simulink model "MATE_SimpleRLC"  (R2024b)
settings: Solver=FixedStepDiscrete  StartTime=0.0  StopTime=0.03  FixedStep=Ts  RelTol=1e-3  AbsTol=1e-2
PostLoadFcn:
  | Ts = 30e-6;
InitFcn:
  | Ts = 30e-6;
StartFcn:
  | Ts=100e-6;
undefined symbols (not defined in the file): MATE, MATE1ph, MATERT, simetran
libraries: fl_lib x17, nesl_utility x9, ee_lib x4, simetranss x2
settings Model: ARTEMISmethode_block_infos=$$__separator__$$  ModifiedByFormat=Kyle  Creator=Kyle Diller  LastModifiedBy=Kyle
settings SolverCC: AutoScaleAbsTol=off  AlgebraicLoopSolver=TrustRegion
settings DataIOCC: SaveFormat=Array  SignalLoggingSaveFormat=ModelDataLogs  ReturnWorkspaceOutputs=off  TimeSaveName=t  OutputSaveName=y  SignalLoggingName=sigsOut
settings OptimizationCC: BlockReduction=off  BooleanDataType=off  ExpressionDepthLimit=2147483647  InitFltsAndDblsToZero=on  LifeSpan=inf
settings DebuggingCC: AlgebraicLoopMsg=none  SaveWithParameterizedLinksMsg=none  UnderspecifiedInitializationDetection=Classic  MergeDetectMultiDrivingBlocksExec=none  SignalResolutionControl=TryResolveAllWithWarning  MultiTaskDSMMsg=warning  MultiTaskCondExecSysMsg=none  FcnCallInpInsideContextMsg=warning  UnconnectedInputMsg=warning  UnconnectedOutputMsg=warning  UnconnectedLineMsg=warning  AllowSymbolicDim=off  StateNameClashWarn=warning  SFUnexpectedBacktrackingDiag=warning  SFNoUnconditionalDefaultTransitionDiag=warning  SFExecutionAtInitializationDiag=none  ArithmeticOperatorsInVariantConditions=warning
settings HardwareCC: ProdBitPerPointer=32  ProdBitPerSizeT=32  ProdBitPerPtrDiffT=32  ProdLargestAtomicFloat=None  ProdIntDivRoundTo=Undefined  ProdEndianess=Unspecified  ProdWordSize=32  ProdHWDeviceType=32-bit Generic  TargetUnknown=on
settings ModelReferenceCC: EnableRefExpFcnMdlSchedulingChecks=on  PropagateSignalLabelsOutOfModel=off
settings SFSimCC: SimUseLocalCustomCode=off  CustomCodeUndefinedFunction=UseInterfaceOnly
settings RTWCC: TemplateMakefile=grt_unix.tmf  RTWUseLocalCustomCode=off  GPUComputeCapability=3.5
settings CodeAppCC: StateflowObjectComments=on
settings GRTTargetCC: TargetFcnLib=ansi_tfl_tmw.mat  TargetLangStandard=C89/C90 (ANSI)  CombineOutputUpdateFcns=off  GRTInterface=on
settings ConfigComp: CovMetricSettings=dw  CovSaveCumulativeToWorkspaceVar=on  CovSaveSingleToWorkspaceVar=on  CovExternalEMLEnable=off
settings SimscapeCC: SimscapeNormalizeSystem=off

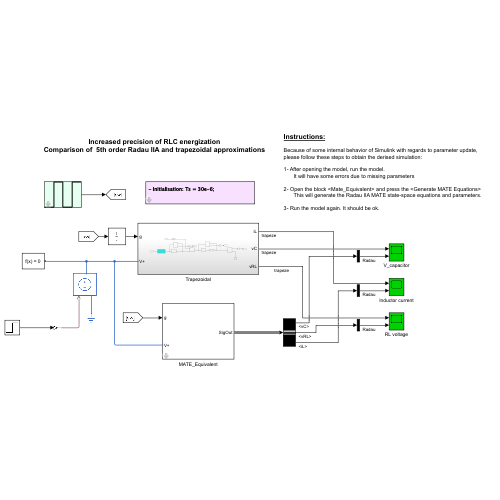
[thumbnail: Simulink's stored preview of the top-level diagram]
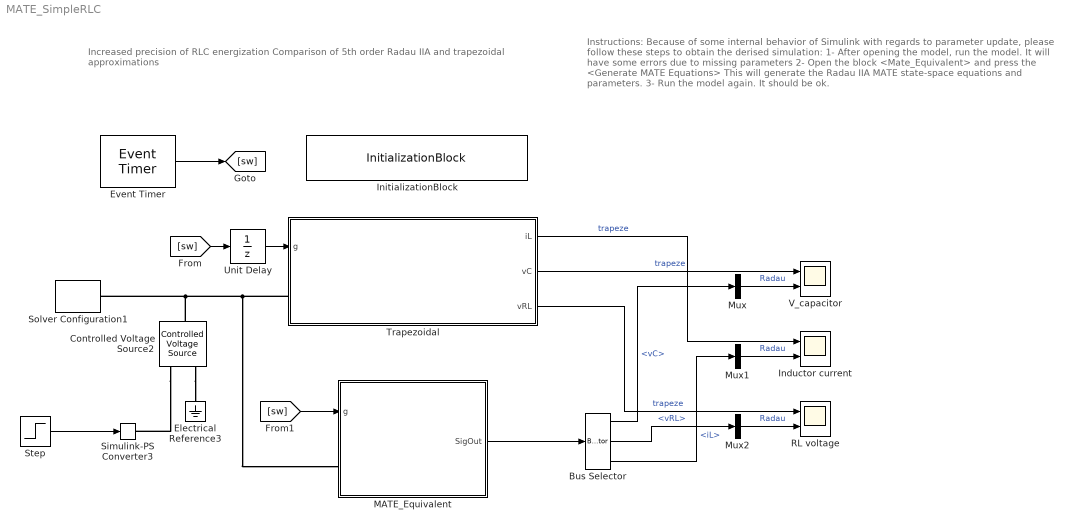
== system MATE_SimpleRLC ==
  note: Instructions:
      |
      | Because of some internal behavior of Simulink with regards to parameter update,
      | please follow these steps to obtain the derised simulation:
      |
      | 1- After opening the model, run the model.
      | It will have some errors due to missing parameters
      |
      | 2- Open the block <Mate_Equivalent> and press the <Generate MATE Equations>
      | This will generate the Radau IIA MATE state-space equations and parameters.
      |
      | 3- Run the model again. It should be ok.
  note: Increased precision of RLC energization
      | Comparison of  5th order Radau IIA and trapezoidal approximations
  Bus Selector : BusSelector  OutputSignals=vC,vRL,iL
  Controlled Voltage Source2 : fl_lib/Electrical/Electrical Sources/Controlled Voltage Source
  Electrical Reference3 : fl_lib/Electrical/Electrical Elements/Electrical Reference
  Event Timer : simetranss/Usefulls/Event Timer  Tag=RTEcontrol_s38shd7k88  is=0 (off)  t=[0.01 0.02 0.03 0.04 ]  Tmax=0.07  Ts=Ts
  Inductor current : Scope  NumInputPorts=2
  InitializationBlock : simetranss/Usefulls/InitializationBlock  InitVar=Ts = 30e-6;  prel=off  posl=on  inif=on
  MATE_Equivalent : Subsystem  mask(MATE object){MATE=MATE, MATERT=MATERT, subsys='MATE_SimpleRLC/Trapezoidal', discmeth=5th order accurate fully-implicit three-stage Runge-Kutta formula (Radau IIA), Tsx=Ts}
      mask prompts: MATE "General MATE data structure name"; MATERT "MATE S-function parameter"; subsys "Reference subsystem for MATE"; discmeth "Discretization"; Tsx "Sample time (s)"
      mask help: The MATE Object contains the MATE solver for mixed nodal and state-space equation of the MATE solution. This is a beta block.
      mask TypeOptions discmeth: Backward Euler | Trapezoidal |  5th order accurate fully-implicit three-stage Runge-Kutta formula (Radau IIA)
      mask DialogControl Control2 Prompt: Generate MATE equations
      mask DialogControl Control2 Callback:
      | block=gcb;
      | maskObj = Simulink.Mask.get(block); % get mask handle
      | Ts = get_param(block, 'value@Tsx'); % retrieve value for Vrated
      | sub = get_param(block, 'value@subsys'); % retrieve value for Vmin_p
      | dd = get_param(block, 'value@discmeth'); % retrieve value for Vmin_p
      | if dd==3
      |     dd=5;
      | end
      | %Tss=get_param(block,'Ts')
      | [MATE, MATERT]= MakeMate2(sub , dd, Ts);
      | assignin("base","MATE",MATE);
      | assignin("base","MATERT",MATERT);
  Mux : Mux  Inputs=1
  Mux1 : Mux  Inputs=1
  Mux2 : Mux  Inputs=1
  RL voltage : Scope  NumInputPorts=2
  Simulink-PS Converter3 : nesl_utility/Simulink-PS Converter  PhysicalDomain=network_engine_domain  SubClassName=ps_input  LeftPortType=input  RightPortType=output  PseudoPeriodic=off  Frequencies=[]  NoiseDistribution=none  NoiseParameters=[]  Unit=1  AffineConversion=off  FilteringAndDerivatives=provide  SimscapeFilterOrder=1  InputFilterTimeConstant=0.001  UdotUserProvided=0
  Solver Configuration1 : nesl_utility/Solver Configuration  PhysicalDomain=network_engine_domain  SubClassName=solver  LeftPortType=input  RightPortType=generic  Tones=[]  Harmonics=[]  SimulateNoise=off  Profile=off  UseLocalSampling=off  EnableSwitchedLinearOptims=on  FrequencyDomain=off  UseCCode=off  RelTol=0.001  AbsTol=1e-06  MinStep=1e-09  ToWorkspace=off  RevertToSquareIcSolve=off  NumHomotopyIterations=100  PhasorMode=off  PhasorModeNumHarmonics=1  ConsistencySolver=NEWTON_FTOL  IndexReductionMethod=DerivativeReplacement  DoDC=off  ResidualTolerance=1e-09  ConsistencyTolSource=GLOBAL  ConsistencyAbsTol=0.001  ConsistencyRelTol=0.001  ConsistencyTolFactor=0.001  UseLocalSolver=on  LocalSolverChoice=NE_TRAPEZOIDAL_ADVANCER  ResolveIndetEquations=on  FunctionEvalNumThread=1  LocalSolverSampleTime=Ts  DoFixedCost=on  MaxNonlinIter=1  MaxModeIter=2  ComputeImpulses=on  ImpulseIterations=2  LinearAlgebra=auto  LinearAlgebraNumThread=0  EquationFormulation=NE_TIME_EF  DelaysMemoryBudget=1024  AutomaticFiltering=on  FilteringTimeConstant=0.001  PartitionStorageMethod=AS_NEEDED  PartitionMemoryBudget=1024  PartitionMethod=ROBUST  MultibodyUseLocalSolver=off  MultibodyLocalSolverChoice=ODE1  MultibodyLocalSolverSampleTime=0.001
  Step : Step  Time=1e-3  SampleTime=0
  Trapezoidal : Subsystem
  Unit Delay : UnitDelay  SampleTime=Ts  HasFrameUpgradeWarning=on
  V_capacitor : Scope  NumInputPorts=2
  wires:
  MATE_Equivalent/1(SigOut) -> Bus Selector/1
  [sw] -> Unit Delay/1
  [sw] -> MATE_Equivalent/1(g)
  Event Timer/1 -> [sw]
  Trapezoidal/3(vRL) -> RL voltage/1  "trapeze"
  Trapezoidal/1(iL) -> Inductor current/1  "trapeze"
  Bus Selector/3 -> Mux1/1  "<iL>"
  Trapezoidal/2(vC) -> V_capacitor/1  "trapeze"
  Bus Selector/1 -> Mux/1  "<vC>"
  Bus Selector/2 -> Mux2/1  "<vRL>"
  Step/1 -> Simulink-PS Converter3/1
  Unit Delay/1 -> Trapezoidal/1(g)
  Mux/1 -> V_capacitor/2  "Radau"
  Mux1/1 -> Inductor current/2  "Radau"
  Mux2/1 -> RL voltage/2  "Radau"
  connections:
  Solver Configuration1/RConn1 -- Trapezoidal/LConn1 -- MATE_Equivalent/LConn1 -- Controlled Voltage Source2/LConn1
  Controlled Voltage Source2/RConn2 -- Electrical Reference3/LConn1
  Controlled Voltage Source2/RConn1 -- Simulink-PS Converter3/RConn1

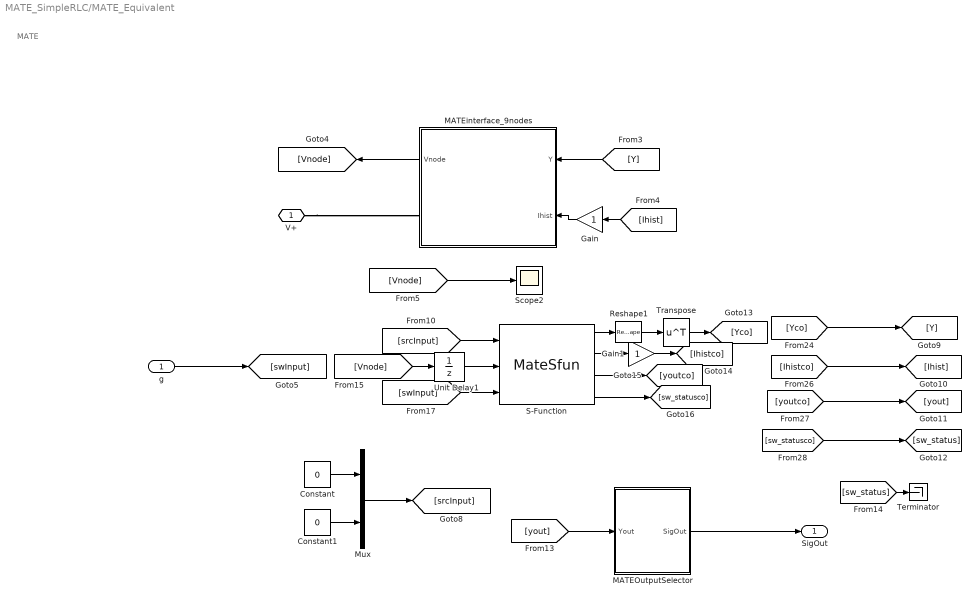
== system MATE_SimpleRLC/MATE_Equivalent ==
  note: MATE
  g : Inport
  Constant : Constant  Value=0
  Constant1 : Constant  Value=0
  Gain : Gain
  Gain1 : Gain
  MATEOutputSelector : Subsystem
  MATEinterface_9nodes : Subsystem
  Mux : Mux  Inputs=2
  Reshape1 : Reshape  OutputDimensionality=Customize  OutputDimensions=[MATE.NumberOfNodes,MATE.NumberOfNodes]
  S-Function : S-Function  FunctionName=MateSfun  Parameters="MATERT.sizes,MATERT.As  ,MATERT.Bs,MATERT.Cs,MATERT.Ds,MATERT.Rsw,MATERT.SwType,MATERT.DISC,MATERT.h,MATERT.U0,MATERT.X0,MATERT.SwitchVf"  SFunctionDeploymentMode=off  EnableBusSupport=off
  Scope2 : Scope
  Terminator : Terminator
  Transpose : Math  Operator=transpose
  Unit Delay1 : UnitDelay  SampleTime=Ts  HasFrameUpgradeWarning=on
  V+ : PMIOPort  Side=Left
  SigOut : Outport
  wires:
  MATEOutputSelector/1(SigOut) -> SigOut/1
  [Vnode] -> Scope2/1
  Mux/1 -> [srcInput]
  g/1 -> [swInput]
  [Yco] -> [Y]
  S-Function/4 -> [sw_statusco]
  [Ihist] -> Gain/1
  [srcInput] -> S-Function/1
  [Ihistco] -> [Ihist]
  Unit Delay1/1 -> S-Function/2
  [swInput] -> S-Function/3
  Reshape1/1 -> Transpose/1
  [Y] -> MATEinterface_9nodes/1(Y)
  [sw_status] -> Terminator/1
  Transpose/1 -> [Yco]
  [yout] -> MATEOutputSelector/1(Yout)
  S-Function/3 -> [youtco]
  [Vnode] -> Unit Delay1/1
  [youtco] -> [yout]
  S-Function/2 -> Gain1/1
  MATEinterface_9nodes/1(Vnode) -> [Vnode]
  S-Function/1 -> Reshape1/1
  [sw_statusco] -> [sw_status]
  Gain/1 -> MATEinterface_9nodes/2(Ihist)
  Gain1/1 -> [Ihistco]
  Constant/1 -> Mux/1
  Constant1/1 -> Mux/2
  connections:
  V+/RConn1 -- MATEinterface_9nodes/RConn1

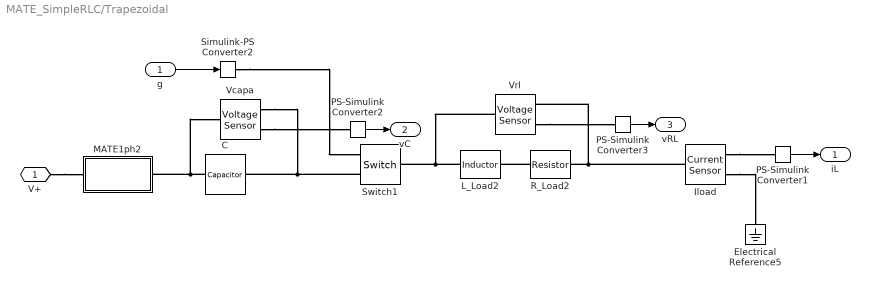
== system MATE_SimpleRLC/Trapezoidal ==
  g : Inport
  C : fl_lib/Electrical/Electrical Elements/Capacitor  c=1e-6 F  r=0 Ohm  g=0 1/Ohm  i_specify=off  i_priority=None  i=0 A  i_nominal_specify=off  i_nominal_value=1  i_nominal_unit=A  v_specify=on  v_priority=None  v=0 V  v_nominal_specify=off  v_nominal_value=1  v_nominal_unit=V  vc_specify=off  vc_priority=High  vc=0 V  vc_nominal_specify=off  vc_nominal_value=1  vc_nominal_unit=V
      settings: AttributesFormatString=%<c> %<c_unit>
  Electrical Reference5 : fl_lib/Electrical/Electrical Elements/Electrical Reference
  Iload : fl_lib/Electrical/Electrical Sensors/Current Sensor
  L_Load2 : fl_lib/Electrical/Electrical Elements/Inductor  l=3e-3 H  r=0 Ohm  g=0 1/Ohm  i_specify=on  i_priority=None  i=0 A  i_nominal_specify=off  i_nominal_value=1  i_nominal_unit=A  v_specify=off  v_priority=None  v=0 V  v_nominal_specify=off  v_nominal_value=1  v_nominal_unit=V  i_L_specify=off  i_L_priority=High  i_L=0 A  i_L_nominal_specify=off  i_L_nominal_value=1  i_L_nominal_unit=A
      settings: AttributesFormatString=%<l> %<l_unit>
  MATE1ph2 : Subsystem  AncestorBlock=simetran/MATE1ph  mask(MATE Node (1ph)){bn=1, conty=Single-Phase, it=auto, Rse=1e-4, Rsh=1e9}
      mask prompts: bn "MATE node number"; conty "Connection"; it "Interface type"; Rse "Series resistance (Ohms)"; Rsh "Shunt resistance (Ohms)"
      mask help:
      | MATE interface for single phase SimScape model.
      |
      | This block is used to interface a MATE reduced set of block to a main circuit.
      | 'MATE' port must be connected toward the MATE reduced network.
      | 'Main' port must be connected toward the main (unreduced) network)
      settings: AttributesFormatString=# %<bn>
      mask TypeOptions conty: Single-Phase | 3-phase SLD | 3-phase expended
      mask TypeOptions it: auto | Thevenin | Norton
  PS-Simulink Converter1 : nesl_utility/PS-Simulink Converter  PhysicalDomain=network_engine_domain  SubClassName=ps_output  LeftPortType=input  RightPortType=output  PseudoPeriodic=off  Frequencies=[]  VectorFormat=inherit  Unit=inherit  AffineConversion=off
  PS-Simulink Converter2 : nesl_utility/PS-Simulink Converter  PhysicalDomain=network_engine_domain  SubClassName=ps_output  LeftPortType=input  RightPortType=output  PseudoPeriodic=off  Frequencies=[]  VectorFormat=inherit  Unit=inherit  AffineConversion=off
  PS-Simulink Converter3 : nesl_utility/PS-Simulink Converter  PhysicalDomain=network_engine_domain  SubClassName=ps_output  LeftPortType=input  RightPortType=output  PseudoPeriodic=off  Frequencies=[]  VectorFormat=inherit  Unit=inherit  AffineConversion=off
  R_Load2 : fl_lib/Electrical/Electrical Elements/Resistor  R=2 Ohm  i_specify=off  i_priority=None  i=0 A  i_nominal_specify=off  i_nominal_value=1  i_nominal_unit=A  v_specify=off  v_priority=None  v=0 V  v_nominal_specify=off  v_nominal_value=1  v_nominal_unit=V
      settings: AttributesFormatString=%<R> %<R_unit>
  Simulink-PS Converter2 : nesl_utility/Simulink-PS Converter  PhysicalDomain=network_engine_domain  SubClassName=ps_input  LeftPortType=input  RightPortType=output  PseudoPeriodic=off  Frequencies=[]  NoiseDistribution=none  NoiseParameters=[]  Unit=1  AffineConversion=off  FilteringAndDerivatives=provide  SimscapeFilterOrder=1  InputFilterTimeConstant=0.001  UdotUserProvided=0
  Switch1 : fl_lib/Electrical/Electrical Elements/Switch  R_closed=0.01 Ohm  G_open=1e-8 1/Ohm  Threshold=0.5  i_specify=off  i_priority=None  i=0 A  i_nominal_specify=off  i_nominal_value=1  i_nominal_unit=A  v_specify=off  v_priority=None  v=0 V  v_nominal_specify=off  v_nominal_value=1  v_nominal_unit=V
  Vcapa : fl_lib/Electrical/Electrical Sensors/Voltage Sensor
  Vrl : fl_lib/Electrical/Electrical Sensors/Voltage Sensor
  V+ : PMIOPort  Side=Left
  iL : Outport
  vC : Outport  Port=2
  vRL : Outport  Port=3
  wires:
  PS-Simulink Converter2/1 -> vC/1
  PS-Simulink Converter1/1 -> iL/1
  g/1 -> Simulink-PS Converter2/1
  PS-Simulink Converter3/1 -> vRL/1
  connections:
  C/RConn1 -- Vcapa/LConn1 -- MATE1ph2/RConn1
  Vcapa/RConn2 -- Switch1/RConn2 -- C/LConn1
  Iload/RConn1 -- PS-Simulink Converter1/LConn1
  Vcapa/RConn1 -- PS-Simulink Converter2/LConn1
  V+/RConn1 -- MATE1ph2/LConn1
  Simulink-PS Converter2/RConn1 -- Switch1/RConn1
  L_Load2/LConn1 -- Vrl/LConn1 -- Switch1/LConn1
  Iload/RConn2 -- Electrical Reference5/LConn1
  Iload/LConn1 -- Vrl/RConn2 -- R_Load2/RConn1
  R_Load2/LConn1 -- L_Load2/RConn1
  Vrl/RConn1 -- PS-Simulink Converter3/LConn1

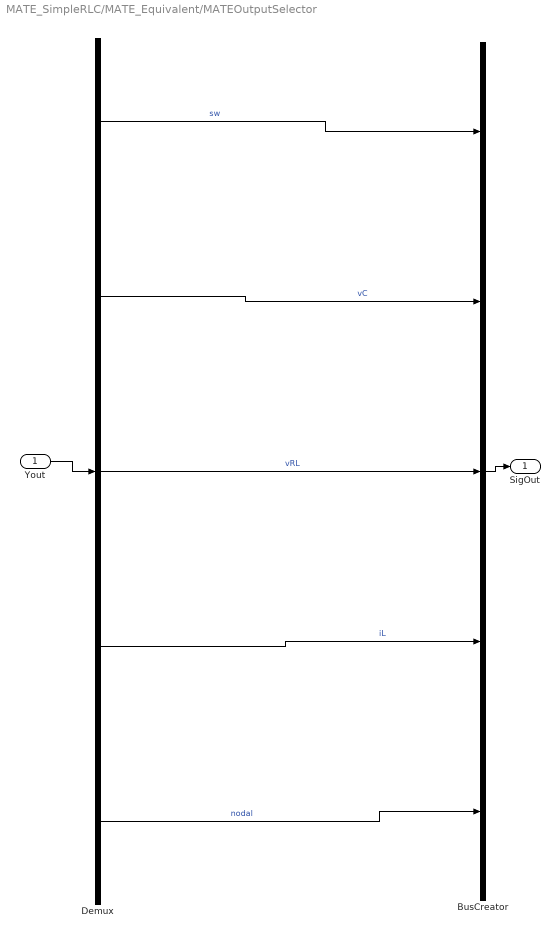
== system MATE_SimpleRLC/MATE_Equivalent/MATEOutputSelector ==
  Yout : Inport
  BusCreator : BusCreator  Inputs=5
  Demux : Demux  Outputs=5
  SigOut : Outport
  wires:
  Yout/1 -> Demux/1
  BusCreator/1 -> SigOut/1
  Demux/1 -> BusCreator/1  "sw"
  Demux/2 -> BusCreator/2  "vC"
  Demux/3 -> BusCreator/3  "vRL"
  Demux/4 -> BusCreator/4  "iL"
  Demux/5 -> BusCreator/5  "nodal"

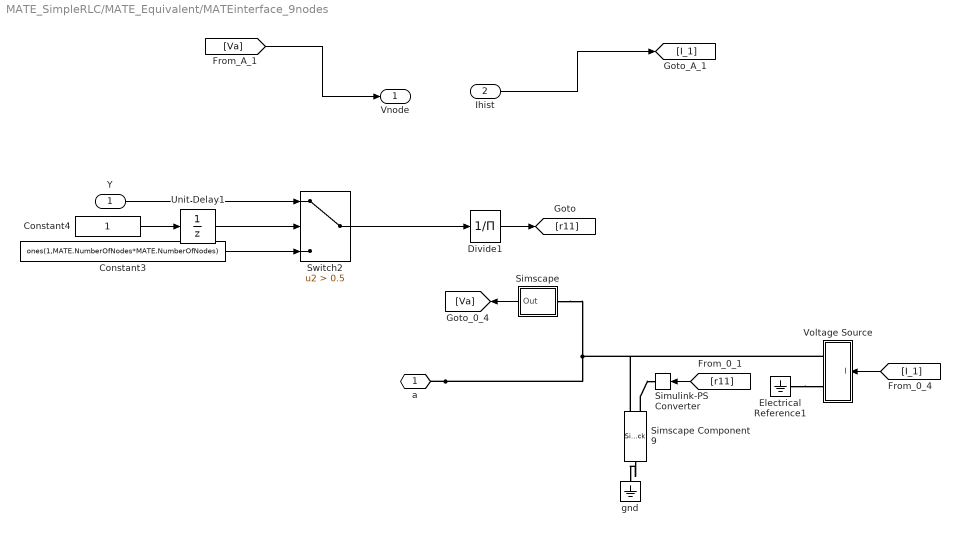
== system MATE_SimpleRLC/MATE_Equivalent/MATEinterface_9nodes ==
  Y : Inport
  Ihist : Inport  Port=2
  Constant3 : Constant  Value=ones(1,MATE.NumberOfNodes*MATE.NumberOfNodes)  SampleTime=Ts
  Constant4 : Constant  SampleTime=Ts
  Divide1 : Product  Inputs=/
  Electrical Reference1 : fl_lib/Electrical/Electrical Elements/Electrical Reference
  Simscape : Subsystem
      mask Display: disp('V')
  Simscape Component9 : SimscapeComponentBlock  SourceFile=variable_resistor_unlimited  ComponentPath=variable_resistor_unlimited  ComponentVariants="[\"variable_resistor_unlimited\"]"  ComponentVariantNames="[\"variable_resistor_unlimited\"]"  ClassName=variable_resistor_unlimited  SchemaVersion=1  R0=0 Ohm  Rmaxp=1e9 Ohm  Rmaxn=-1e9 Ohm  Rminp=1e-9 Ohm  Rminn=-1e-9 Ohm  i_specify=off  i_priority=None  i=0 A  i_nominal_specify=off  i_nominal_value=1  i_nominal_unit=A  v_specify=off  v_priority=None  v=0 V  v_nominal_specify=off  v_nominal_value=1  v_nominal_unit=V
      settings: CopyFcn=simscape.engine.sli.internal.componentblockcallback(gcbh,'COPY')  PreCopyFcn=simscape.engine.sli.internal.componentblockcallback(gcbh,'PRECOPY')  PreDeleteFcn=simscape.engine.sli.internal.componentblockcallback(gcbh,'PREDELETE')  InternalSimscapePortConfiguration="{\"Bottom\":[],\"Left\":[{\"id\":\"R\",\"label\":\"R\",\"type\":\"input\"},{\"id\":\"p\",\"label\":\"+\",\"type\":\"foundation.electrical.electrical\"}],\"Right\":[{\"id\":\"n\",\"label\":\"-\",\"type\":\"foundation.electrical.electrical\"}],\"Top\":[]}"
      mask Type: Variable Resistor
  Simulink-PS Converter : nesl_utility/Simulink-PS Converter  PhysicalDomain=network_engine_domain  SubClassName=ps_input  LeftPortType=input  RightPortType=output  PseudoPeriodic=off  Frequencies=[]  NoiseDistribution=none  NoiseParameters=[]  Unit=1  AffineConversion=off  FilteringAndDerivatives=provide  SimscapeFilterOrder=1  InputFilterTimeConstant=0.001  UdotUserProvided=0
  Switch2 : Switch  Criteria=u2 > Threshold  Threshold=0.5  SaturateOnIntegerOverflow=off  InputSameDT=off
  Unit Delay1 : UnitDelay  SampleTime=Ts  HasFrameUpgradeWarning=on
  Voltage Source : Subsystem
  gnd : fl_lib/Electrical/Electrical Elements/Electrical Reference
  a : PMIOPort  Side=Right
  Vnode : Outport  VectorParamsAs1DForOutWhenUnconnected=off
  wires:
  Constant3/1 -> Switch2/3
  Constant4/1 -> Unit Delay1/1
  Unit Delay1/1 -> Switch2/2
  Divide1/1 -> [r11]
  Switch2/1 -> Divide1/1
  [r11] -> Simulink-PS Converter/1
  Y/1 -> Switch2/1
  [I_1] -> Voltage Source/1(I)
  Simscape/1(Out) -> [Va]
  [Va] -> Vnode/1
  Ihist/1 -> [I_1]
  connections:
  Simscape Component9/LConn1 -- Simulink-PS Converter/RConn1
  Simscape Component9/RConn1 -- gnd/LConn1
  Electrical Reference1/LConn1 -- Voltage Source/RConn2
  a/RConn1 -- Simscape/LConn1 -- Voltage Source/RConn1 -- Simscape Component9/LConn2

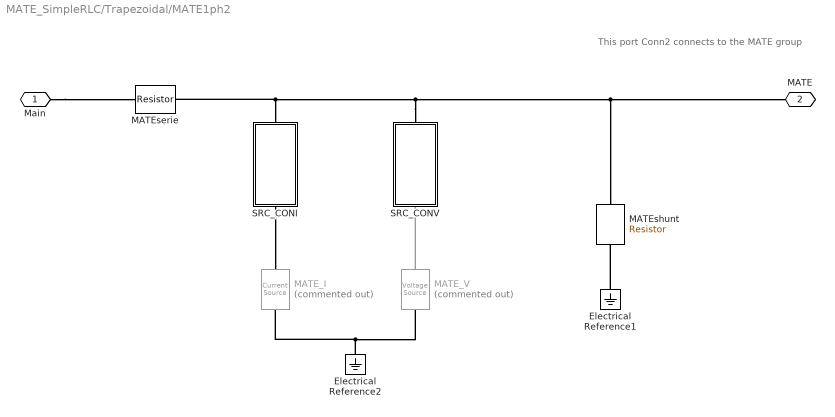
== system MATE_SimpleRLC/Trapezoidal/MATE1ph2 ==
  note: This port Conn2 connects to the MATE group
  Electrical Reference1 : fl_lib/Electrical/Electrical Elements/Electrical Reference
  Electrical Reference2 : fl_lib/Electrical/Electrical Elements/Electrical Reference
  MATE_I : ee_lib/Sources/Current Source  Commented=on  dc_current=0 A  ac_current=0 A  ac_shift=0 rad  ac_frequency=60 Hz  noise_mode=ee.enum.sources.noise.Disabled  PSD=0 A^2/Hz  sample_time=1e-3 s  repeatability=ee.enum.sources.repeatability.NotRepeatable  user_seed=0  auto_seed=153380492  i_specify=off  i_priority=None  i=0 A  i_nominal_specify=off  i_nominal_value=1  i_nominal_unit=A  v_specify=off  v_priority=None  v=0 V  v_nominal_specify=off  v_nominal_value=1  v_nominal_unit=V
  MATE_V : ee_lib/Sources/Voltage Source  Commented=on  dc_voltage=0 V  ac_voltage=0 V  ac_shift=0 rad  ac_frequency=1 Hz  noise_mode=ee.enum.sources.noise.Disabled  PSD=0 V^2/Hz  sample_time=1e-3 s  repeatability=ee.enum.sources.repeatability.NotRepeatable  user_seed=0  auto_seed=3646982598  i_specify=off  i_priority=None  i=0 A  i_nominal_specify=off  i_nominal_value=1  i_nominal_unit=A  v_specify=off  v_priority=None  v=0 V  v_nominal_specify=off  v_nominal_value=1  v_nominal_unit=V
  MATEserie : ee_lib/Passive/Resistor  R=Rse Ohm  enable_R_tol=ee.enum.toleranceApplication.none  R_tol=5  tol_distribution=ee.enum.toleranceDistribution.uniform  nSigma=4  enable_operating_limits=ee.enum.enable.no  operating_limit_action=ee.enum.passive.reportOpLim.warn  power_rating=1 W  max_working_voltage=100 V  noise_mode=ee.enum.sources.noise.Disabled  Tdevice=25 degC  sample_time=1e-3 s  repeatability=ee.enum.ic.repeatability.notRepeatable  user_seed=0  auto_seed=4011470453  fault_action=simscape.enum.assert.action.none  t_fault=1 s  power_derating_T1=70 degC  power_derating_T2=155 degC  operating_temperature_range_vec=[-50, 150] degC  alpha=3.93e-3 1/K  Tmeas=25 degC  thermal_mass=100 J/K  temperature_specify=off  temperature_priority=High  temperature=298.15 K  temperature_nominal_specify=off  temperature_nominal_value=1  temperature_nominal_unit=K
  MATEshunt : ee_lib/Passive/Resistor  R=Rsh Ohm  enable_R_tol=ee.enum.toleranceApplication.none  R_tol=5  tol_distribution=ee.enum.toleranceDistribution.uniform  nSigma=4  enable_operating_limits=ee.enum.enable.no  operating_limit_action=ee.enum.passive.reportOpLim.warn  power_rating=1 W  max_working_voltage=100 V  noise_mode=ee.enum.sources.noise.Disabled  Tdevice=25 degC  sample_time=1e-3 s  repeatability=ee.enum.ic.repeatability.notRepeatable  user_seed=0  auto_seed=2915145293  fault_action=simscape.enum.assert.action.none  t_fault=1 s  power_derating_T1=70 degC  power_derating_T2=155 degC  operating_temperature_range_vec=[-50, 150] degC  alpha=3.93e-3 1/K  Tmeas=25 degC  thermal_mass=100 J/K  temperature_specify=off  temperature_priority=High  temperature=298.15 K  temperature_nominal_specify=off  temperature_nominal_value=1  temperature_nominal_unit=K
  SRC_CONI : Subsystem
  SRC_CONV : Subsystem
  Main : PMIOPort  Side=Left
  MATE : PMIOPort  Port=2  Side=Right
  connections:
  Main/RConn1 -- MATEserie/LConn1
  SRC_CONV/LConn1 -- MATEserie/RConn1 -- SRC_CONI/LConn1 -- MATEshunt/LConn1 -- MATE/RConn1
  Electrical Reference1/LConn1 -- MATEshunt/RConn1
  MATE_V/LConn1 -- SRC_CONV/RConn1
  Electrical Reference2/LConn1 -- MATE_I/RConn1 -- MATE_V/RConn1
  SRC_CONI/RConn1 -- MATE_I/LConn1

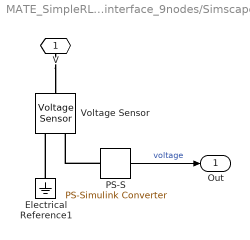
== system MATE_SimpleRLC/MATE_Equivalent/MATEinterface_9nodes/Simscape ==
  Electrical Reference1 : fl_lib/Electrical/Electrical Elements/Electrical Reference
  PS-S : nesl_utility/PS-Simulink Converter  PhysicalDomain=network_engine_domain  SubClassName=ps_output  LeftPortType=input  RightPortType=output  PseudoPeriodic=off  Frequencies=[]  VectorFormat=1-D array  Unit=V  AffineConversion=off
  Voltage Sensor : fl_lib/Electrical/Electrical Sensors/Voltage Sensor
  V : PMIOPort  Side=Left
  Out : Outport  VectorParamsAs1DForOutWhenUnconnected=off
  wires:
  PS-S/1 -> Out/1  "voltage"
  connections:
  PS-S/LConn1 -- Voltage Sensor/RConn1
  V/RConn1 -- Voltage Sensor/LConn1
  Electrical Reference1/LConn1 -- Voltage Sensor/RConn2

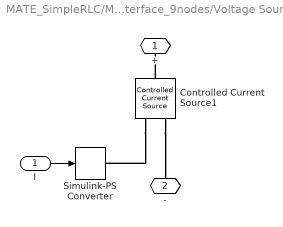
== system MATE_SimpleRLC/MATE_Equivalent/MATEinterface_9nodes/Voltage Source ==
  I : Inport
  Controlled Current Source1 : fl_lib/Electrical/Electrical Sources/Controlled Current Source
  Simulink-PS Converter : nesl_utility/Simulink-PS Converter  PhysicalDomain=network_engine_domain  SubClassName=ps_input  LeftPortType=input  RightPortType=output  PseudoPeriodic=off  Frequencies=[]  NoiseDistribution=none  NoiseParameters=[]  Unit=1  AffineConversion=off  FilteringAndDerivatives=zero  SimscapeFilterOrder=1  InputFilterTimeConstant=.001  UdotUserProvided=0
  + : PMIOPort  Side=Right
  - : PMIOPort  Port=2  Side=Right
  wires:
  I/1 -> Simulink-PS Converter/1
  connections:
  Controlled Current Source1/RConn1 -- Simulink-PS Converter/RConn1
  Controlled Current Source1/RConn2 -- -/RConn1
  Controlled Current Source1/LConn1 -- +/RConn1

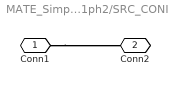
== system MATE_SimpleRLC/Trapezoidal/MATE1ph2/SRC_CONI ==
  Conn1 : PMIOPort  Side=Left
  Conn2 : PMIOPort  Port=2  Side=Right
  connections:
  Conn1/RConn1 -- Conn2/RConn1

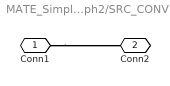
== system MATE_SimpleRLC/Trapezoidal/MATE1ph2/SRC_CONV ==
  Conn1 : PMIOPort  Side=Left
  Conn2 : PMIOPort  Port=2  Side=Right
  connections:
  Conn1/RConn1 -- Conn2/RConn1
